simulink model "tich2sine"  (R2021b)
settings: Solver=VariableStepAuto  StartTime=0.0  StopTime=10.0  RelTol=1e-3
libraries: simulink x2
settings Model: Creator=ryuzuu  LastModifiedBy=ryuzuu

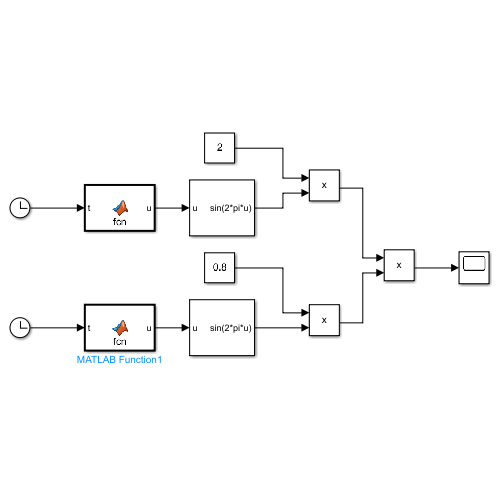
[thumbnail: Simulink's stored preview of the top-level diagram]
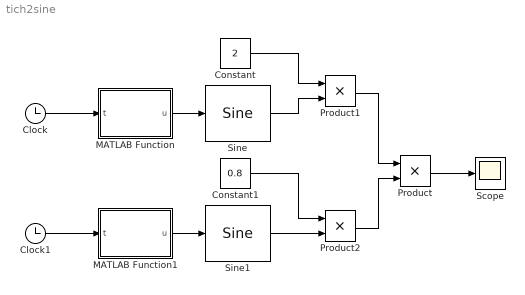
== system tich2sine ==
  Clock : Clock
  Clock1 : Clock
  Constant : Constant  Value=2
  Constant1 : Constant  Value=0.8
  MATLAB Function : MATLAB Function  TreatAsAtomicUnit=on
  MATLAB Function1 : MATLAB Function  TreatAsAtomicUnit=on
  Product : Product
  Product1 : Product
  Product2 : Product
  Scope : Scope
  Sine : simulink/Lookup Tables/Sine  Formula=sin(2*pi*u)  NumDataPoints=(2^5)+1  OutputWordLength=16  InternalRulePriority=Speed
  Sine1 : simulink/Lookup Tables/Sine  Formula=sin(2*pi*u)  NumDataPoints=(2^5)+1  OutputWordLength=16  InternalRulePriority=Speed
  wires:
  Product/1 -> Scope/1
  Clock1/1 -> MATLAB Function1/1(t)
  Sine/1 -> Product1/2
  Constant/1 -> Product1/1
  Sine1/1 -> Product2/2
  Constant1/1 -> Product2/1
  Product1/1 -> Product/1
  Product2/1 -> Product/2
  MATLAB Function/1(u) -> Sine/1
  MATLAB Function1/1(u) -> Sine1/1
  Clock/1 -> MATLAB Function/1(t)

== matlab function tich2sine/MATLAB Function ==
  data: t input; u output
function u = fcn(t)

u = 0.1*t;

== matlab function tich2sine/MATLAB Function1 ==
  data: t input; u output
function u = fcn(t)

u = 0.05*t;
